simulink library "rtwdemo_autosar_csinterface"  (Simulink 7.6)
settings: Solver=ode45  StartTime=0.0  StopTime=10.0  RelTol=1e-3
libraries: rtwlib x1, rtwdemo_autosar_csinterface x1
settings Model: Creator=batserve  LastModifiedBy=batserve

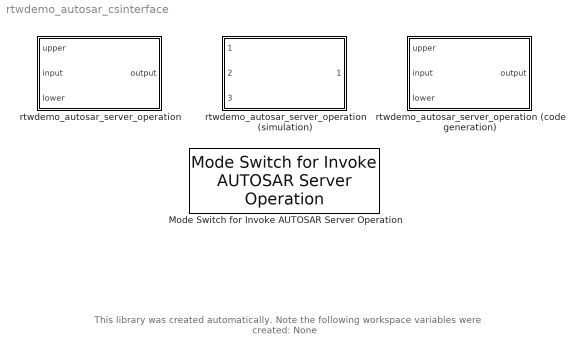
== system rtwdemo_autosar_csinterface ==
  note: This library was created automatically.
      | Note the following workspace variables were created:
      | None
  Mode Switch for Invoke AUTOSAR Server Operation : rtwlib/AUTOSAR/Mode Switch for Invoke AUTOSAR Server Operation  SystemSampleTime=-1  mode=code generation  ShowInLibBrowser=on
  rtwdemo_autosar_server_operation : Subsystem  Tag=AUTOSARConfigSubsystem  BlockChoice=|
      | rtwdemo_autosar_server_operation
      | (code generation)
      settings: TemplateBlock=self
      settings: MemberBlocks=|
      | rtwdemo_autosar_server_operation
      | (code generation),rtwdemo_autosar_server_operation
      | (simulation)
  rtwdemo_autosar_server_operation (code generation) : Subsystem  mask(Invoke AUTOSAR Server Operation){portName=Port, operationPrototype=rtwdemo_autosar_server_operation(IN double upper, IN double input, IN double lower, OUT double output), interfacePath=/rtwdemo_autosar/csinterface, serverType=Application software, showErrorStatus=off, SAMPLETIME=-1, showARPortLabels=off}
      mask prompts: portName "Client port name:"; operationPrototype "Operation prototype:"; interfacePath "Interface path:"; serverType "Server type:"; showErrorStatus "Show error status"; SAMPLETIME "Sample time (-1 for inherited):"; showARPortLabels "Show port labels"
      mask help:
      | Configure AUTOSAR client port to access Basic Software or Application Software Components with an arbitrary number of arguments. You can use this block to generate code for accessing a server port.
      |
      | Specify the type and number of inports and outports in the operation prototype field, in the form: "op(IN uint8 data1, OUT double data2[10])"
      mask init:
      | hblk = gcbh;
      | [maskDisplay, iIsBuiltin,iIsBus,iDtIdx,iWidth,iIsExpr,iDtStr,oIsBuiltin,oIsBus,oDtIdx,oWidth,oIsExpr,oDtStr,tlcStr] = sfun_autosar_clientop_blk( 'configure', gcbh );
      | set_param(hblk, 'MaskDisplay', maskDisplay);
      mask Help: helpview([docroot '/toolbox/ecoder/helptargets.map'], 'autosar_client_op_block');
      mask StyleString: edit,edit,edit,popup(Application software|Basic software),checkbox,edit,checkbox
      mask Display: image(imread('sfun_autosar_clientop.bmp'),'center');
  rtwdemo_autosar_server_operation (simulation) : ModelReference  ModelNameDialog=rtwdemo_autosar_server_operation  SimulationMode=Accelerator  ModelReferenceVersion=1.1  CopyOfModelName=rtwdemo_autosar_server_operation

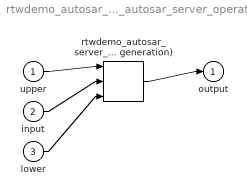
== system rtwdemo_autosar_csinterface/rtwdemo_autosar_server_operation ==
  upper : Inport
  input : Inport  Port=2
  lower : Inport  Port=3
  rtwdemo_autosar_server_operation (code generation) : rtwdemo_autosar_csinterface/rtwdemo_autosar_server_operation (code generation)  SystemSampleTime=-1  portName=Port  operationPrototype=rtwdemo_autosar_server_operation(IN double upper, IN double input, IN double lower, OUT double output)  interfacePath=/rtwdemo_autosar/csinterface  serverType=Application software  showErrorStatus=off  SAMPLETIME=-1  showARPortLabels=off
  output : Outport
  wires:
  upper/1 -> rtwdemo_autosar_server_operation (code generation)/1
  input/1 -> rtwdemo_autosar_server_operation (code generation)/2
  lower/1 -> rtwdemo_autosar_server_operation (code generation)/3
  rtwdemo_autosar_server_operation (code generation)/1 -> output/1

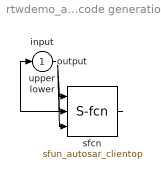
== system rtwdemo_autosar_csinterface/rtwdemo_autosar_server_operation (code generation) ==
  upper : Inport
  input : Inport  Port=2
  lower : Inport  Port=3
  sfcn : S-Function  FunctionName=sfun_autosar_clientop  Parameters=iIsBuiltin, iIsBus, iDtIdx, iDtStr, iWidth, iIsExpr, oIsBuiltin, oIsBus, oDtIdx, oDtStr, oWidth, oIsExpr, tlcStr, SAMPLETIME  EnableBusSupport=off
  output : Outport
  wires:
  upper/1 -> sfcn/1
  input/1 -> sfcn/2
  lower/1 -> sfcn/3
  sfcn/1 -> output/1
